simulink model "compassGaitSim"  (R2013a)
settings: Solver=ode45  StartTime=0.0  StopTime=5.00  FixedStep=0.01  MaxStep=0.02  MinStep=1e-16  RelTol=1e-3
values from neighbouring files (symbols this model uses):
  g = 9.81    [getDynParams.m]
  ground = [-realmax, 0 ... (first row only)    [RunSim.m]    (also in runSim2.m)
  I1 = Is(1)    [ZeroDynCompassGait.m]    (also in getDynParams.m = 0.166979166667; runSim2.m)
  I2 = Is(2)    [ZeroDynCompassGait.m]    (also in getDynParams.m = 0.0419791666667; nomTorque.m = I(2); nomTorqueCG.m = I(2); runSim2.m)
  l1 = ls(1)    [ZeroDynCompassGait.m]    (also in getDynParams.m = 1; runSim2.m)
  l2 = ls(2)    [ZeroDynCompassGait.m]    (also in getDynParams.m = 1; runSim2.m)
  m1 = ms(1)    [ZeroDynCompassGait.m]    (also in getDynParams.m = 0.5; runSim2.m)
  m2 = ms(2)    [ZeroDynCompassGait.m]    (also in getDynParams.m = 0.5; runSim2.m)
  org = endSwingFoot(q(:,end),org)    [RunSim.m]    (also in runSim2.m = [0, 0])
  points = origPoints    [ConstrGui.m]    (also in runSim2.m = constrData(1).points)
undefined symbols (not defined in the file or in its folder): nom_torque_table, t1_0, t1d_0, t2_0, t2d_0
settings Model: CovHTMLOptions=-sRT=1 -aTS=1 -bRG=1 -bTC=1 -hTR=0 -nFC=0 -scm=1 -bcm=1 -xEv=0  Creator=yak  LastModifiedBy=yak
settings SolverCC: MaxConsecutiveMinStep=10
settings DataIOCC: LimitDataPoints=off  OutputOption=SpecifiedOutputTimes  OutputTimes=0:0.01:(timeleft-0.01)
settings DebuggingCC: DiscreteInheritContinuousMsg=none  MultiTaskDSMMsg=warning  MultiTaskCondExecSysMsg=none  FcnCallInpInsideContextMsg=EnableAllAsWarning  StrictBusMsg=None
settings RTWCC: IncludeERTFirstTime=on

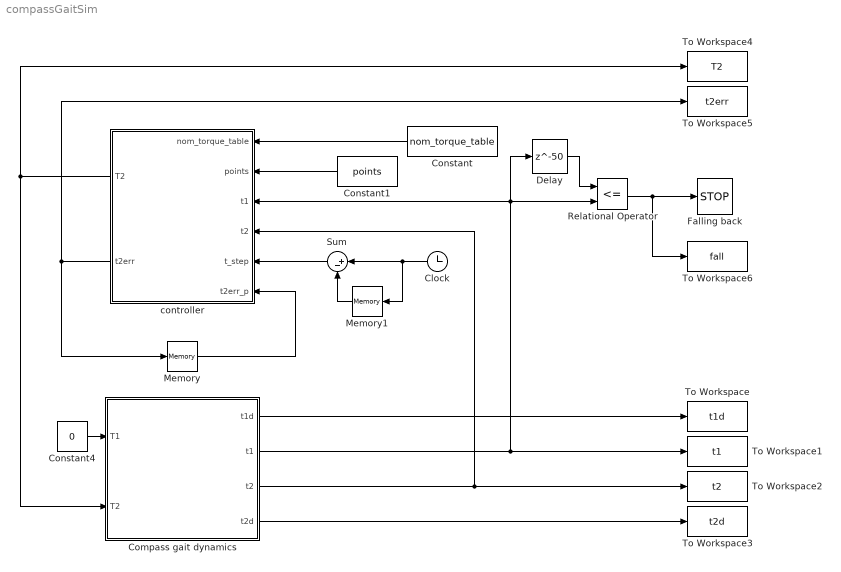
== system compassGaitSim ==
  Clock : Clock
  Compass gait dynamics : Subsystem
  Constant : Constant  Value=nom_torque_table
  Constant1 : Constant  Value=points
  Constant4 : Constant  Value=0
  Delay : Delay  DelayLength=50  InitialCondition=100  SampleTime=0.01
  Falling back : Stop
  Memory : Memory
  Memory1 : Memory  X0=-0.02
  Relational Operator : RelationalOperator  Operator=<=  OutDataTypeStr=boolean  ZeroCross=off
  Sum : Sum  Inputs=|+-
  To Workspace : ToWorkspace  VariableName=t1d  SampleTime=-1
  To Workspace1 : ToWorkspace  VariableName=t1  SampleTime=-1
  To Workspace2 : ToWorkspace  VariableName=t2  SampleTime=-1
  To Workspace3 : ToWorkspace  VariableName=t2d  SampleTime=-1
  To Workspace4 : ToWorkspace  VariableName=T2  SampleTime=-1
  To Workspace5 : ToWorkspace  VariableName=t2err  SampleTime=-1
  To Workspace6 : ToWorkspace  VariableName=fall  SampleTime=-1
      settings: MaxDataPoints=1
  controller : MATLAB Function  TreatAsAtomicUnit=on
  wires:
  controller/1(T2) -> To Workspace4/1, Compass gait dynamics/2(T2)
  Compass gait dynamics/1(t1d) -> To Workspace/1
  Compass gait dynamics/2(t1) -> To Workspace1/1, Delay/1, controller/3(t1), Relational Operator/2
  Compass gait dynamics/3(t2) -> To Workspace2/1, controller/4(t2)
  Compass gait dynamics/4(t2d) -> To Workspace3/1
  Constant4/1 -> Compass gait dynamics/1(T1)
  Constant/1 -> controller/1(nom_torque_table)
  Delay/1 -> Relational Operator/1
  Relational Operator/1 -> To Workspace6/1, Falling back/1
  controller/2(t2err) -> To Workspace5/1, Memory/1
  Memory/1 -> controller/6(t2err_p)
  Clock/1 -> Sum/1, Memory1/1
  Sum/1 -> controller/5(t_step)
  Memory1/1 -> Sum/2
  Constant1/1 -> controller/2(points)

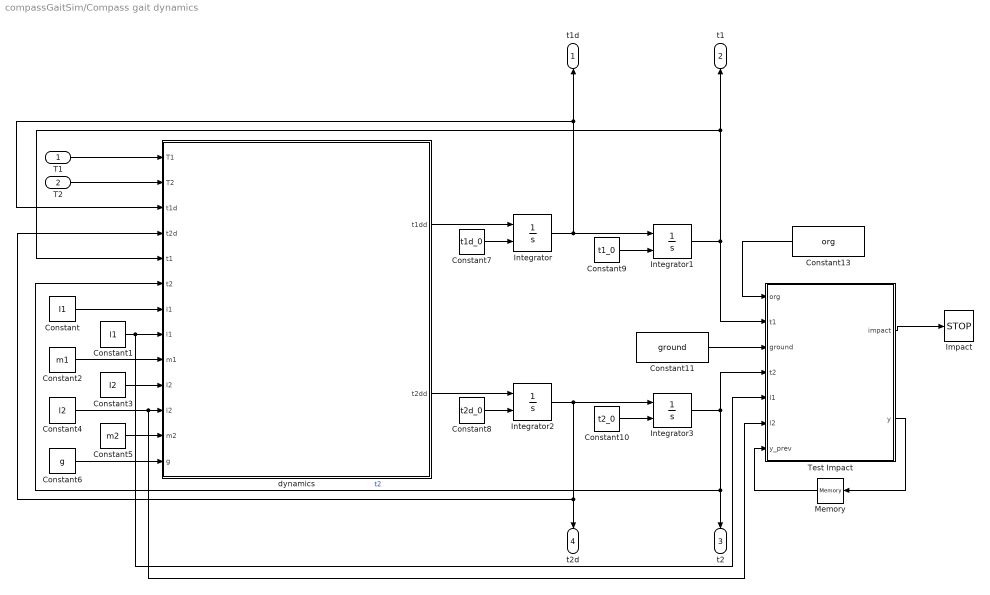
== system compassGaitSim/Compass gait dynamics ==
  T1 : Inport
  T2 : Inport  Port=2
  Constant : Constant  Value=I1
  Constant1 : Constant  Value=l1
  Constant10 : Constant  Value=t2_0
  Constant11 : Constant  Value=ground
  Constant13 : Constant  Value=org
  Constant2 : Constant  Value=m1
  Constant3 : Constant  Value=I2
  Constant4 : Constant  Value=l2
  Constant5 : Constant  Value=m2
  Constant6 : Constant  Value=g
  Constant7 : Constant  Value=t1d_0
  Constant8 : Constant  Value=t2d_0
  Constant9 : Constant  Value=t1_0
  Impact : Stop
  Integrator{,1..3} (4 alike) : Integrator  InitialConditionSource=external
  Memory : Memory
  Test Impact : MATLAB Function  TreatAsAtomicUnit=on
  dynamics : MATLAB Function  TreatAsAtomicUnit=on
  t1d : Outport
  t1 : Outport  Port=2
  t2 : Outport  Port=3
  t2d : Outport  Port=4
  wires:
  T1/1 -> dynamics/1(T1)
  T2/1 -> dynamics/2(T2)
  dynamics/1(t1dd) -> Integrator/1
  Integrator/1 -> t1d/1, dynamics/3(t1d), Integrator1/1
  Integrator2/1 -> t2d/1, dynamics/4(t2d), Integrator3/1
  Integrator3/1 -> t2/1, dynamics/6(t2), Test Impact/4(t2)  "t2"
  Integrator1/1 -> Test Impact/2(t1), dynamics/5(t1), t1/1
  Constant2/1 -> dynamics/9(m1)
  Constant/1 -> dynamics/7(I1)
  Constant1/1 -> Test Impact/5(l1), dynamics/8(l1)
  Constant3/1 -> dynamics/10(I2)
  Constant4/1 -> Test Impact/6(l2), dynamics/11(l2)
  Constant5/1 -> dynamics/12(m2)
  Constant6/1 -> dynamics/13(g)
  Constant7/1 -> Integrator/2
  Constant9/1 -> Integrator1/2
  dynamics/2(t2dd) -> Integrator2/1
  Test Impact/1(impact) -> Impact/1
  Constant8/1 -> Integrator2/2
  Constant10/1 -> Integrator3/2
  Constant11/1 -> Test Impact/3(ground)
  Test Impact/2(y) -> Memory/1
  Memory/1 -> Test Impact/7(y_prev)
  Constant13/1 -> Test Impact/1(org)

== matlab function compassGaitSim/controller ==
  data: nom_torque_table input; points input; t1 input; t2 input; t_step input; T2 output; t2err output; t2err_p input
function [T2, t2err] = ...
    controller(nom_torque_table, points, t1, t2, t_step, t2err_p)
%#codegen

%% Feed-forward Zero Dynamics
% Linearly interpolate from pre-computed values.
i = find(t1 <= nom_torque_table(:,1), 1, 'last');
if isempty(i)
    T2 = 0;
else 
    i = i(1);
    if i < size(nom_torque_table,1)
        ths = nom_torque_table(i:i+1,1);
        us = nom_torque_table(i:i+1,2);
        T2 = (us(2)-us(1))/(ths(2)-ths(1)) * (t1-ths(1)) + us(1);
    else
        T2 = 0;
    end
end

%% Simple PD feedback controller
% This is used to correct any disturbance from the zero dynamics
K_p = 0;%1000;
K_d = 0;%100;

% Calculate desired th2
t = (t1 - points(1,1)) / (points(end,1) - points(1,1));
t(t>1) = 1;
t(t<0) = 0;
t2_des = 0;
n = size(points, 1) - 1;
for i = 0 : n
    t2_des = t2_des + nchoosek(n,i) * (1-t)^(n-i) * t^i * points(i+1,2);
end

t2err = t2_des - t2;
% Ensure error is within 1 rotation
t2err = mod(t2err, 2*pi);   
% Ensure error is in the range [-pi pi]
if t2err > pi
    t2err = -(2*pi - t2err);
elseif t2err < -pi
    t2err = 2*pi - t2err;
end
% Calculate derivative of error
t2ed = t2err - t2err_p;
% Account for discontinuity
t2ed(t2ed > pi) = t2ed - pi;
t2ed(t2ed < -pi) = t2ed + pi;
t2ed = t2ed / t_step;

T2 = T2 + K_p*t2err + K_d*t2ed;
end

== matlab function compassGaitSim/Compass gait dynamics/dynamics ==
  data: T1 input; t1dd output; T2 input; t1d input; t2d input; t1 input; t2 input; t2dd output; I1 input; l1 input; m1 input; I2 input; l2 input; m2 input; g input
function [t1dd, t2dd] = compassGaitDynamics(T1, T2, t1d, t2d, t1, t2, ...
    I1, l1, m1, I2, l2, m2, g)
%#codegen

c1 = cos(t1);
c2 = cos(t2);
s2 = sin(t2);
c12 = cos(t1 + t2);


% Equations in terms of T1 and T2 are derived, then the solution in terms
% of the angle accelerations have been pre-solved. The output is below.
t1dd = (4*I2*T1 - 4*I2*T2 + T1*l2^2*m2 - T2*l2^2*m2 - ...
    c1*g*l1*l2^2*m2^2 - 2*I2*c1*g*l1*m1 - 4*I2*c1*g*l1*m2 - ...
    2*T2*c2*l1*l2*m2 + (l1*l2^3*m2^2*s2*t1d^2)/2 + ...
    (l1*l2^3*m2^2*s2*t2d^2)/2 + 2*I2*l1*l2*m2*s2*t1d^2 + ...
    2*I2*l1*l2*m2*s2*t2d^2 - (c1*g*l1*l2^2*m1*m2)/2 + ...
    c2*l1^2*l2^2*m2^2*s2*t1d^2 + c2*c12*g*l1*l2^2*m2^2 + ...
    l1*l2^3*m2^2*s2*t1d*t2d + 4*I2*l1*l2*m2*s2*t1d*t2d)/ ...
    (- c2^2*l1^2*l2^2*m2^2 + l1^2*l2^2*m2^2 + ...
    4*I2*l1^2*m2 + I1*l2^2*m2 + 4*I1*I2);

t2dd = -(4*I2*T1 - 4*I1*T2 - 4*I2*T2 + T1*l2^2*m2 - 4*T2*l1^2*m2 - ...
    T2*l2^2*m2 - c1*g*l1*l2^2*m2^2 + 2*c12*g*l1^2*l2*m2^2 - ...
    2*I2*c1*g*l1*m1 - 4*I2*c1*g*l1*m2 + 2*I1*c12*g*l2*m2 + ...
    2*T1*c2*l1*l2*m2 - 4*T2*c2*l1*l2*m2 + (l1*l2^3*m2^2*s2*t1d^2)/2 + ...
    2*l1^3*l2*m2^2*s2*t1d^2 + (l1*l2^3*m2^2*s2*t2d^2)/2 + ...
    2*I1*l1*l2*m2*s2*t1d^2 + 2*I2*l1*l2*m2*s2*t1d^2 + ...
    2*I2*l1*l2*m2*s2*t2d^2 - (c1*g*l1*l2^2*m1*m2)/2 + ...
    2*c2*l1^2*l2^2*m2^2*s2*t1d^2 + c2*l1^2*l2^2*m2^2*s2*t2d^2 - ...
    2*c1*c2*g*l1^2*l2*m2^2 + c2*c12*g*l1*l2^2*m2^2 + ...
    l1*l2^3*m2^2*s2*t1d*t2d + 4*I2*l1*l2*m2*s2*t1d*t2d + ...
    2*c2*l1^2*l2^2*m2^2*s2*t1d*t2d - c1*c2*g*l1^2*l2*m1*m2)/(- ...
    c2^2*l1^2*l2^2*m2^2 + l1^2*l2^2*m2^2 + 4*I2*l1^2*m2 + I1*l2^2*m2 + ...
    4*I1*I2);

end

== matlab function compassGaitSim/Compass gait dynamics/Test Impact ==
  data: org input; t1 input; ground input; impact output; t2 input; l1 input; l2 input; y_prev input; y output
function [impact, y] = ...
    isImpact(org, t1, ground, t2, l1, l2, y_prev)
%#codegen

impact = false;
y=0;
height=0;

% Impact when the foot descends onto the ground after it has passed the
% midpoint of the swing phase.

% Calculate x and y position of foot.
x = org(1) + l1*cos(t1) + l2*cos(t1+t2);
y = org(2) + l1*sin(t1) + l2*sin(t1+t2);

% Find height of ground underneath foot.
ind = find(x>ground(:,1), 1, 'last');
height = ground(ind,2);
height = height(1);

% Impact only if on falling edge and if stance leg is behind swing leg.
if y <= height && y_prev > height && t2 > -pi
    impact = true;
end

end
